simulink model "exp3_1_formation_linear"  (R2020b)
settings: Solver=VariableStepAuto  StartTime=0  StopTime=50  RelTol=1e-3
values from neighbouring files (symbols this model uses):
  g = 9.8    [run_exp1.m]    (also in run_exp2.m; run_exp3_1.m; run_exp3_2.m)
  Ixx = 0.114    [run_exp1.m]    (also in run_exp2.m; run_exp3_1.m; run_exp3_2.m)
  Iyy = 0.114    [run_exp1.m]    (also in run_exp2.m; run_exp3_1.m; run_exp3_2.m)
  Izz = 0.158    [run_exp1.m]    (also in run_exp2.m; run_exp3_1.m; run_exp3_2.m)
  k_F = 6.11*10^(-8)*3600/(4*pi^2)    (= 5.57165188849e-06)    [run_exp1.m]    (also in run_exp2.m; run_exp3_1.m; run_exp3_2.m)
  k_M = 1.5*10^(-9)*3600/(4*pi^2)    (= 1.36783597917e-07)    [run_exp1.m]    (also in run_exp2.m; run_exp3_1.m; run_exp3_2.m)
  k_m = 20    [run_exp1.m]    (also in run_exp2.m; run_exp3_1.m; run_exp3_2.m)
  kat_i = 0.05    [run_exp2.m]    (also in run_exp3_1.m; run_exp3_2.m)
  kat_p = 1    [run_exp2.m]    (also in run_exp3_1.m; run_exp3_2.m)
  kct_d = 1    [run_exp2.m]    (also in run_exp3_1.m; run_exp3_2.m)
  kct_i = 0.05    [run_exp2.m]    (also in run_exp3_1.m; run_exp3_2.m)
  kct_p = 1    [run_exp2.m]    (also in run_exp3_1.m; run_exp3_2.m)
  kd_phi = 4000    [run_exp1.m]    (also in run_exp2.m; run_exp3_1.m; run_exp3_2.m)
  kd_psi = 4000    [run_exp1.m]    (also in run_exp2.m; run_exp3_1.m; run_exp3_2.m)
  kd_theta = 4000    [run_exp1.m]    (also in run_exp2.m; run_exp3_1.m; run_exp3_2.m)
  kd_x = 1.0    (= 1)    [run_exp1.m]    (also in run_exp2.m; run_exp3_1.m; run_exp3_2.m)
  kd_y = 1.0    (= 1)    [run_exp1.m]    (also in run_exp2.m; run_exp3_1.m; run_exp3_2.m)
  kd_z = 2.0    (= 2)    [run_exp1.m]    (also in run_exp2.m; run_exp3_1.m; run_exp3_2.m)
  ki_x = 3e-4    (= 0.0003)    [run_exp1.m]    (also in run_exp2.m; run_exp3_1.m; run_exp3_2.m = 0.01)
  ki_y = 3e-4    (= 0.0003)    [run_exp1.m]    (also in run_exp2.m; run_exp3_1.m; run_exp3_2.m = 0.01)
  ki_z = 1e-6    (= 1e-06)    [run_exp1.m]    (also in run_exp2.m; run_exp3_1.m; run_exp3_2.m)
  kp_phi = 2000    [run_exp1.m]    (also in run_exp2.m; run_exp3_1.m; run_exp3_2.m)
  kp_psi = 800    [run_exp1.m]    (also in run_exp2.m; run_exp3_1.m; run_exp3_2.m)
  kp_theta = 2000    [run_exp1.m]    (also in run_exp2.m; run_exp3_1.m; run_exp3_2.m)
  kp_x = 0.5    [run_exp1.m]    (also in run_exp2.m; run_exp3_1.m; run_exp3_2.m = 1)
  kp_y = 0.5    [run_exp1.m]    (also in run_exp2.m; run_exp3_1.m; run_exp3_2.m = 1)
  kp_z = 1.2    [run_exp1.m]    (also in run_exp2.m; run_exp3_1.m; run_exp3_2.m)
  L = 0.2    [run_exp1.m]    (also in run_exp2.m; run_exp3_1.m; run_exp3_2.m)
  m = 0.5    [run_exp1.m]    (also in run_exp2.m; run_exp3_1.m; run_exp3_2.m)
  R = 0.5    [run_exp3_1.m]    (also in run_exp3_2.m = formation(4))
  state_track = [0,0,0,0 ... (first row only)    [run_exp2.m]    (also in run_exp3_1.m)
  y1_init = 0    [run_exp3_1.m]    (also in run_exp3_2.m)
  y2_init = R    (= 0.5)    [run_exp3_1.m]    (also in run_exp3_2.m = 5)
  y3_init = -R    (= -0.5)    [run_exp3_1.m]    (also in run_exp3_2.m = -5)
libraries: pid_lib x12, shared6dof x3, dspindex x1, dspswit3 x1
(part 2 of 2)

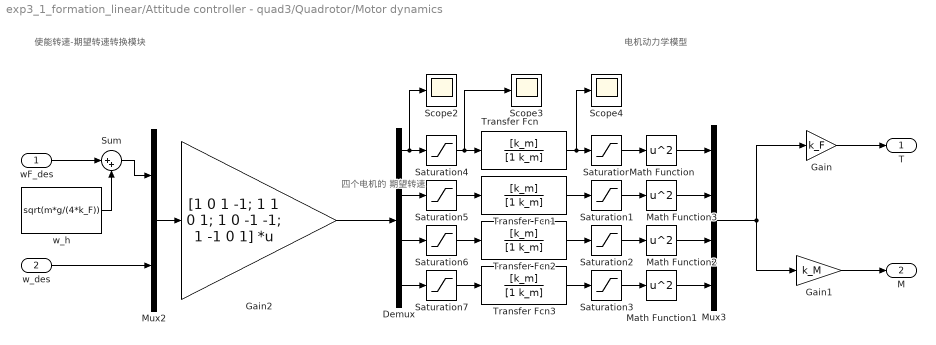
== system exp3_1_formation_linear/Attitude controller - quad3/Quadrotor/Motor dynamics ==
  note: 四个电机的
      | 期望转速
  note: 电机动力学模型
  note: 使能转速-期望转速转换模块
  wF_des : Inport
  w_des : Inport  Port=2
  Demux : Demux
  Gain : Gain  Gain=k_F
  Gain1 : Gain  Gain=k_M
  Gain2 : Gain  Gain=[1 0 1 -1; 1 1 0 1; 1 0 -1 -1; 1 -1 0 1]  Multiplication=Matrix(K*u) (u vector)
  Math Function{,1..3} (4 alike) : Math  Operator=square  SaturateOnIntegerOverflow=on
  Mux2 : Mux  Inputs=2
  Mux3 : Mux
  Saturation{,1..7} (8 alike) : Saturate  UpperLimit=7800*2*pi/60  LowerLimit=1200*2*pi/60
  Scope2 : Scope
  Scope3 : Scope
  Scope4 : Scope
  Sum : Sum  Inputs=|++
  Transfer Fcn{,1..3} (4 alike) : TransferFcn  Numerator=[k_m]  Denominator=[1 k_m]
  w_h : Constant  Value=sqrt(m*g/(4*k_F))
  T : Outport
  M : Outport  Port=2
  wires:
  Mux2/1 -> Gain2/1
  Sum/1 -> Mux2/1
  w_h/1 -> Sum/2
  Gain/1 -> T/1
  Mux3/1 -> Gain1/1, Gain/1
  Gain2/1 -> Demux/1
  Gain1/1 -> M/1
  wF_des/1 -> Sum/1
  Math Function/1 -> Mux3/1
  Math Function3/1 -> Mux3/2
  Math Function2/1 -> Mux3/3
  Math Function1/1 -> Mux3/4
  Transfer Fcn3/1 -> Saturation3/1
  Transfer Fcn/1 -> Scope4/1, Saturation/1
  Transfer Fcn1/1 -> Saturation1/1
  Transfer Fcn2/1 -> Saturation2/1
  Saturation/1 -> Math Function/1
  Saturation3/1 -> Math Function1/1
  Saturation2/1 -> Math Function2/1
  Saturation1/1 -> Math Function3/1
  w_des/1 -> Mux2/2
  Saturation6/1 -> Transfer Fcn2/1
  Saturation7/1 -> Transfer Fcn3/1
  Saturation4/1 -> Scope3/1, Transfer Fcn/1
  Saturation5/1 -> Transfer Fcn1/1
  Demux/1 -> Scope2/1, Saturation4/1
  Demux/2 -> Saturation5/1
  Demux/3 -> Saturation6/1
  Demux/4 -> Saturation7/1

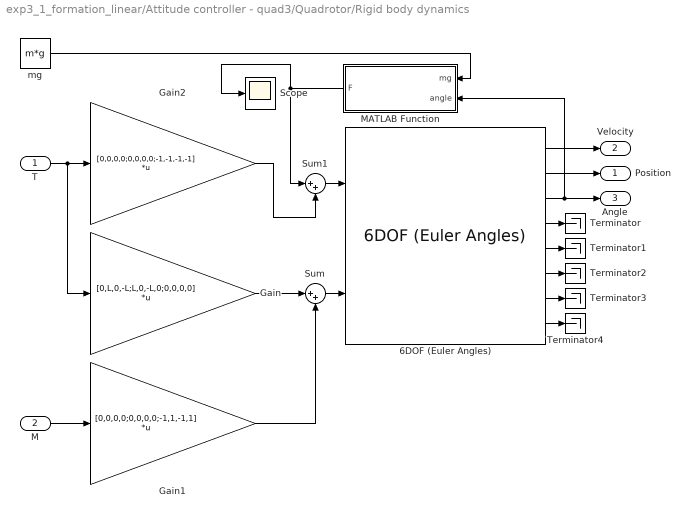
== system exp3_1_formation_linear/Attitude controller - quad3/Quadrotor/Rigid body dynamics ==
  T : Inport
  M : Inport  Port=2
  6DOF (Euler Angles) : shared6dof/6DOF (Euler Angles)  units=Metric (MKS)  mtype=Fixed  rep=Euler Angles  xme_0=[0 y3_init 0]  Vm_0=[0 0 0]  eul_0=[0 0 0]  pm_0=[0 0 0]  mass_0=m  mass_e=0.5  mass_f=2.0  inertia=[Ixx,0,0; 0,Iyy,0; 0,0,Izz]  inertia_e=eye(3)  inertia_f=2*eye(3)  k_quat=1.0  vre_flag=on  abi_flag=off  aMode=0  xme_statename=''  Vm_statename=''  eul_statename=''  quat_statename=''  pm_statename=''  mass_statename=''
      settings: SourceProductBaseCode=AE,PW,MT,UV,VE,VP
  Gain : Gain  Gain=[0,L,0,-L;L,0,-L,0;0,0,0,0]  Multiplication=Matrix(K*u) (u vector)
  Gain1 : Gain  Gain=[0,0,0,0;0,0,0,0;-1,1,-1,1]  Multiplication=Matrix(K*u) (u vector)
  Gain2 : Gain  Gain=[0,0,0,0;0,0,0,0;-1,-1,-1,-1]  Multiplication=Matrix(K*u) (u vector)
  MATLAB Function : MATLAB Function  TreatAsAtomicUnit=on
  Scope : Scope
  Sum : Sum  Inputs=|++
  Sum1 : Sum  Inputs=|++
  Terminator{,1..4} (5 alike) : Terminator
  mg : Constant  Value=m*g
  Position : Outport
  Velocity : Outport  Port=2
  Angle : Outport  Port=3
  wires:
  6DOF (Euler Angles)/1 -> Velocity/1
  T/1 -> Gain/1, Gain2/1
  6DOF (Euler Angles)/3 -> MATLAB Function/2(angle), Angle/1
  6DOF (Euler Angles)/2 -> Position/1
  Gain1/1 -> Sum/2
  Gain/1 -> Sum/1
  Sum/1 -> 6DOF (Euler Angles)/2
  M/1 -> Gain1/1
  Sum1/1 -> 6DOF (Euler Angles)/1
  Gain2/1 -> Sum1/2
  6DOF (Euler Angles)/4 -> Terminator/1
  6DOF (Euler Angles)/5 -> Terminator1/1
  6DOF (Euler Angles)/6 -> Terminator2/1
  6DOF (Euler Angles)/7 -> Terminator3/1
  6DOF (Euler Angles)/8 -> Terminator4/1
  mg/1 -> MATLAB Function/1(mg)
  MATLAB Function/1(F) -> Sum1/1, Scope/1

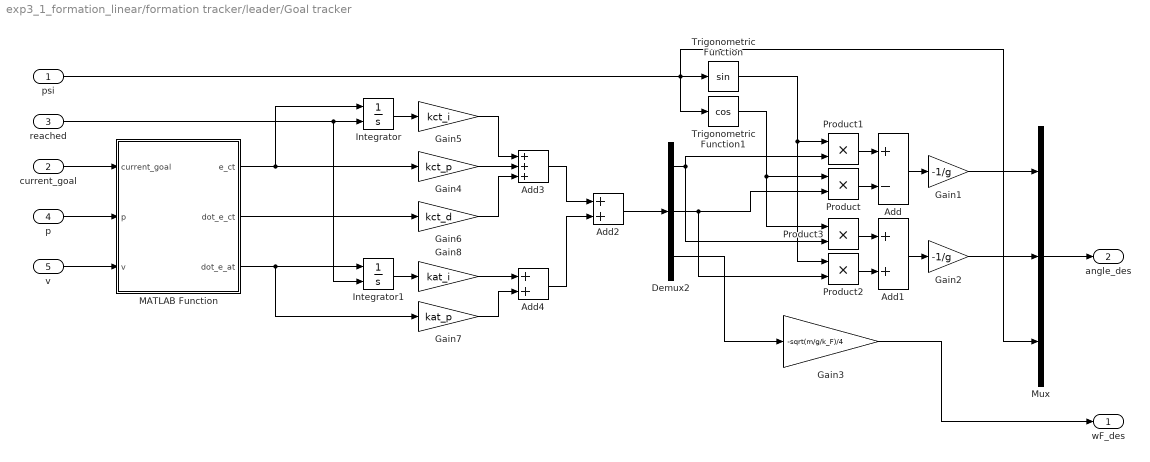
== system exp3_1_formation_linear/formation tracker/leader/Goal tracker ==
  psi : Inport
  current_goal : Inport  Port=2
  reached : Inport  Port=3
  p : Inport  Port=4
  v : Inport  Port=5
  Add : Sum  Inputs=+-
  Add1 : Sum
  Add2 : Sum
  Add3 : Sum  Inputs=+++
  Add4 : Sum
  Demux2 : Demux  Outputs=3
  Gain1 : Gain  Gain=-1/g
  Gain2 : Gain  Gain=-1/g
  Gain3 : Gain  Gain=-sqrt(m/g/k_F)/4
  Gain4 : Gain  Gain=kct_p
  Gain5 : Gain  Gain=kct_i
  Gain6 : Gain  Gain=kct_d
  Gain7 : Gain  Gain=kat_p
  Gain8 : Gain  Gain=kat_i
  Integrator : Integrator  ExternalReset=rising
  Integrator1 : Integrator  ExternalReset=rising
  MATLAB Function : MATLAB Function  TreatAsAtomicUnit=on
  Mux : Mux  Inputs=3
  Product{,1..3} (4 alike) : Product
  Trigonometric Function : Trigonometry
  Trigonometric Function1 : Trigonometry  Operator=cos
  wF_des : Outport
  angle_des : Outport  Port=2
  wires:
  Mux/1 -> angle_des/1
  Gain2/1 -> Mux/2
  Add4/1 -> Add2/2
  Add2/1 -> Demux2/1
  Trigonometric Function1/1 -> Product3/1, Product/1
  MATLAB Function/1(e_ct) -> Integrator/1, Gain4/1
  Demux2/1 -> Product3/2, Product1/2
  psi/1 -> Mux/3, Trigonometric Function1/1, Trigonometric Function/1
  Gain6/1 -> Add3/3
  Add3/1 -> Add2/1
  Product2/1 -> Add1/2
  Trigonometric Function/1 -> Product2/1, Product1/1
  reached/1 -> Integrator1/2, Integrator/2
  Product/1 -> Add/2
  Gain1/1 -> Mux/1
  Demux2/2 -> Product2/2, Product/2
  Demux2/3 -> Gain3/1
  Product3/1 -> Add1/1
  Add/1 -> Gain1/1
  v/1 -> MATLAB Function/3(v)
  Product1/1 -> Add/1
  MATLAB Function/3(dot_e_at) -> Gain7/1, Integrator1/1
  Integrator/1 -> Gain5/1
  Gain5/1 -> Add3/1
  Gain8/1 -> Add4/1
  Integrator1/1 -> Gain8/1
  Gain7/1 -> Add4/2
  Gain4/1 -> Add3/2
  Add1/1 -> Gain2/1
  current_goal/1 -> MATLAB Function/1(current_goal)
  MATLAB Function/2(dot_e_ct) -> Gain6/1
  p/1 -> MATLAB Function/2(p)
  Gain3/1 -> wF_des/1

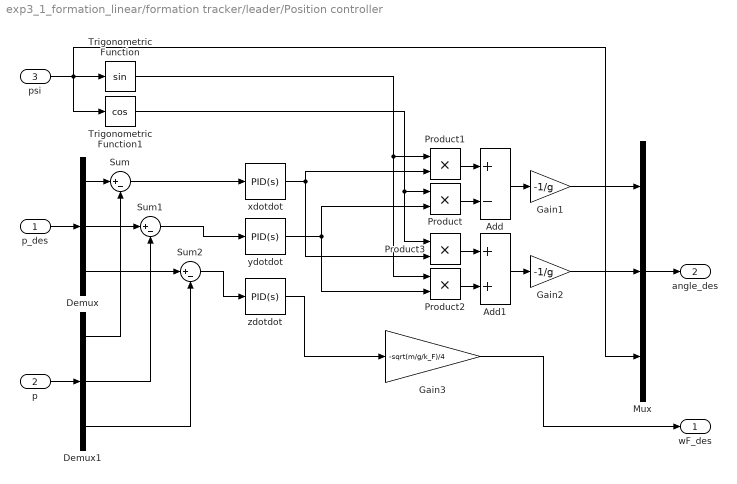
== system exp3_1_formation_linear/formation tracker/leader/Position controller ==
  p_des : Inport
  p : Inport  Port=2
  psi : Inport  Port=3
  Add : Sum  Inputs=+-
  Add1 : Sum
  Demux : Demux  Outputs=3
  Demux1 : Demux  Outputs=3
  Gain1 : Gain  Gain=-1/g
  Gain2 : Gain  Gain=-1/g
  Gain3 : Gain  Gain=-sqrt(m/g/k_F)/4
  Mux : Mux  Inputs=3
  Product{,1..3} (4 alike) : Product
  Sum : Sum  Inputs=|+-
  Sum1 : Sum  Inputs=|+-
  Sum2 : Sum  Inputs=|+-
  Trigonometric Function : Trigonometry
  Trigonometric Function1 : Trigonometry  Operator=cos
  xdotdot : pid_lib/PID Controller  Controller=PID  Form=Parallel  TimeDomain=Continuous-time  UseExternalTs=off  SampleTime=-1  IntegratorMethod=Forward Euler  FilterMethod=Forward Euler  ControllerParametersSource=internal  P=kp_x  I=ki_x  D=kd_x  UseFilter=on  N=100  TunerSelectOption=Transfer Function Based (PID Tuner App)  InitialConditionSource=internal  InitialConditionForIntegrator=0  InitialConditionForFilter=0  DifferentiatorICPrevScaledInput=0  ExternalReset=none  TrackingMode=off  Kt=1  LimitOutput=off  SatLimitsSource=internal  UpperSaturationLimit=inf  LowerSaturationLimit=-inf  LinearizeAsGain=on  AntiWindupMode=none  Kb=1  POutMin=[]  POutMax=[]  IOutMin=[]  IOutMax=[]  DOutMin=[]  DOutMax=[]  NOutMin=[]  NOutMax=[]  SumOutMin=[]  SumOutMax=[]  SaturationOutMin=[]  SaturationOutMax=[]  PParamMin=[]  PParamMax=[]  IParamMin=[]  IParamMax=[]  DParamMin=[]  DParamMax=[]  NParamMin=[]  NParamMax=[]  KbParamMin=[]  KbParamMax=[]  KtParamMin=[]  KtParamMax=[]  KbOutMin=[]  KbOutMax=[]  KtOutMin=[]  KtOutMax=[]  IntegratorOutMin=[]  IntegratorOutMax=[]  FilterOutMin=[]  FilterOutMax=[]  SumI1OutMin=[]  SumI1OutMax=[]  SumI2OutMin=[]  SumI2OutMax=[]  SumI3OutMin=[]  SumI3OutMax=[]  SumI4OutMin=[]  SumI4OutMax=[]  SumDOutMin=[]  SumDOutMax=[]  DifferentiatorOutMin=[]  DifferentiatorOutMax=[]  FilterDiffOutCoefMin=[]  FilterDiffOutCoefMax=[]  ReciprocalOutMin=[]  ReciprocalOutMax=[]  SumDenOutMin=[]  SumDenOutMax=[]  SumNumOutMin=[]  SumNumOutMax=[]  DivideOutMin=[]  DivideOutMax=[]  UdiffTsProdOutMin=[]  UdiffTsProdOutMax=[]  NTsProdOutMin=[]  NTsProdOutMax=[]  UintegralTsProdOutMin=[]  UintegralTsProdOutMax=[]  UngainTsProdOutMin=[]  UngainTsProdOutMax=[]  IntegratorContinuousStateAttributes=''  IntegratorStateMustResolveToSignalObject=off  IntegratorRTWStateStorageClass=Auto  FilterContinuousStateAttributes=''  FilterStateMustResolveToSignalObject=off  FilterRTWStateStorageClass=Auto  ParallelPVariant=InternalParameters  IdealPVariant=Disabled  IVariant=InternalParameters  DVariant=InternalParameters  IntegratorVariant=Continuous  SatVariant=Disabled  AWVariant=Passthrough  PCopyVariant=Disabled  TRVariant=Disabled  FdbkBlocksVariant=Forward  IdealPFdbkVariant=Disabled  SatFdbkVariant=Disabled  DerivativeFilterVariant=ContFilter  NVariant=InternalParameters  NCopyVariant=Disabled  FilterICVariant=InternalICsFilter  IntegratorICVariant=InternalICs  ExternalResetVariant=Disabled  TRSumVariant=Passthrough  SumFdbkVariant=Disabled  SumVariant=Sum_PID  TsampFilterVariant=InternalTs  TsampNgainVariant=Passthrough  TsampIntegralVariant=Passthrough  ExternalSaturationOutDataTypeStr=Inherit: Same as second input
  ydotdot : pid_lib/PID Controller  Controller=PID  Form=Parallel  TimeDomain=Continuous-time  UseExternalTs=off  SampleTime=-1  IntegratorMethod=Forward Euler  FilterMethod=Forward Euler  ControllerParametersSource=internal  P=kp_y  I=ki_y  D=kd_y  UseFilter=on  N=100  TunerSelectOption=Transfer Function Based (PID Tuner App)  InitialConditionSource=internal  InitialConditionForIntegrator=0  InitialConditionForFilter=0  DifferentiatorICPrevScaledInput=0  ExternalReset=none  TrackingMode=off  Kt=1  LimitOutput=off  SatLimitsSource=internal  UpperSaturationLimit=inf  LowerSaturationLimit=-inf  LinearizeAsGain=on  AntiWindupMode=none  Kb=1  POutMin=[]  POutMax=[]  IOutMin=[]  IOutMax=[]  DOutMin=[]  DOutMax=[]  NOutMin=[]  NOutMax=[]  SumOutMin=[]  SumOutMax=[]  SaturationOutMin=[]  SaturationOutMax=[]  PParamMin=[]  PParamMax=[]  IParamMin=[]  IParamMax=[]  DParamMin=[]  DParamMax=[]  NParamMin=[]  NParamMax=[]  KbParamMin=[]  KbParamMax=[]  KtParamMin=[]  KtParamMax=[]  KbOutMin=[]  KbOutMax=[]  KtOutMin=[]  KtOutMax=[]  IntegratorOutMin=[]  IntegratorOutMax=[]  FilterOutMin=[]  FilterOutMax=[]  SumI1OutMin=[]  SumI1OutMax=[]  SumI2OutMin=[]  SumI2OutMax=[]  SumI3OutMin=[]  SumI3OutMax=[]  SumI4OutMin=[]  SumI4OutMax=[]  SumDOutMin=[]  SumDOutMax=[]  DifferentiatorOutMin=[]  DifferentiatorOutMax=[]  FilterDiffOutCoefMin=[]  FilterDiffOutCoefMax=[]  ReciprocalOutMin=[]  ReciprocalOutMax=[]  SumDenOutMin=[]  SumDenOutMax=[]  SumNumOutMin=[]  SumNumOutMax=[]  DivideOutMin=[]  DivideOutMax=[]  UdiffTsProdOutMin=[]  UdiffTsProdOutMax=[]  NTsProdOutMin=[]  NTsProdOutMax=[]  UintegralTsProdOutMin=[]  UintegralTsProdOutMax=[]  UngainTsProdOutMin=[]  UngainTsProdOutMax=[]  IntegratorContinuousStateAttributes=''  IntegratorStateMustResolveToSignalObject=off  IntegratorRTWStateStorageClass=Auto  FilterContinuousStateAttributes=''  FilterStateMustResolveToSignalObject=off  FilterRTWStateStorageClass=Auto  ParallelPVariant=InternalParameters  IdealPVariant=Disabled  IVariant=InternalParameters  DVariant=InternalParameters  IntegratorVariant=Continuous  SatVariant=Disabled  AWVariant=Passthrough  PCopyVariant=Disabled  TRVariant=Disabled  FdbkBlocksVariant=Forward  IdealPFdbkVariant=Disabled  SatFdbkVariant=Disabled  DerivativeFilterVariant=ContFilter  NVariant=InternalParameters  NCopyVariant=Disabled  FilterICVariant=InternalICsFilter  IntegratorICVariant=InternalICs  ExternalResetVariant=Disabled  TRSumVariant=Passthrough  SumFdbkVariant=Disabled  SumVariant=Sum_PID  TsampFilterVariant=InternalTs  TsampNgainVariant=Passthrough  TsampIntegralVariant=Passthrough  ExternalSaturationOutDataTypeStr=Inherit: Same as second input
  zdotdot : pid_lib/PID Controller  Controller=PID  Form=Parallel  TimeDomain=Continuous-time  UseExternalTs=off  SampleTime=-1  IntegratorMethod=Forward Euler  FilterMethod=Forward Euler  ControllerParametersSource=internal  P=kp_z  I=ki_z  D=kd_z  UseFilter=on  N=100  TunerSelectOption=Transfer Function Based (PID Tuner App)  InitialConditionSource=internal  InitialConditionForIntegrator=0  InitialConditionForFilter=0  DifferentiatorICPrevScaledInput=0  ExternalReset=none  TrackingMode=off  Kt=1  LimitOutput=off  SatLimitsSource=internal  UpperSaturationLimit=inf  LowerSaturationLimit=-inf  LinearizeAsGain=on  AntiWindupMode=none  Kb=1  POutMin=[]  POutMax=[]  IOutMin=[]  IOutMax=[]  DOutMin=[]  DOutMax=[]  NOutMin=[]  NOutMax=[]  SumOutMin=[]  SumOutMax=[]  SaturationOutMin=[]  SaturationOutMax=[]  PParamMin=[]  PParamMax=[]  IParamMin=[]  IParamMax=[]  DParamMin=[]  DParamMax=[]  NParamMin=[]  NParamMax=[]  KbParamMin=[]  KbParamMax=[]  KtParamMin=[]  KtParamMax=[]  KbOutMin=[]  KbOutMax=[]  KtOutMin=[]  KtOutMax=[]  IntegratorOutMin=[]  IntegratorOutMax=[]  FilterOutMin=[]  FilterOutMax=[]  SumI1OutMin=[]  SumI1OutMax=[]  SumI2OutMin=[]  SumI2OutMax=[]  SumI3OutMin=[]  SumI3OutMax=[]  SumI4OutMin=[]  SumI4OutMax=[]  SumDOutMin=[]  SumDOutMax=[]  DifferentiatorOutMin=[]  DifferentiatorOutMax=[]  FilterDiffOutCoefMin=[]  FilterDiffOutCoefMax=[]  ReciprocalOutMin=[]  ReciprocalOutMax=[]  SumDenOutMin=[]  SumDenOutMax=[]  SumNumOutMin=[]  SumNumOutMax=[]  DivideOutMin=[]  DivideOutMax=[]  UdiffTsProdOutMin=[]  UdiffTsProdOutMax=[]  NTsProdOutMin=[]  NTsProdOutMax=[]  UintegralTsProdOutMin=[]  UintegralTsProdOutMax=[]  UngainTsProdOutMin=[]  UngainTsProdOutMax=[]  IntegratorContinuousStateAttributes=''  IntegratorStateMustResolveToSignalObject=off  IntegratorRTWStateStorageClass=Auto  FilterContinuousStateAttributes=''  FilterStateMustResolveToSignalObject=off  FilterRTWStateStorageClass=Auto  ParallelPVariant=InternalParameters  IdealPVariant=Disabled  IVariant=InternalParameters  DVariant=InternalParameters  IntegratorVariant=Continuous  SatVariant=Disabled  AWVariant=Passthrough  PCopyVariant=Disabled  TRVariant=Disabled  FdbkBlocksVariant=Forward  IdealPFdbkVariant=Disabled  SatFdbkVariant=Disabled  DerivativeFilterVariant=ContFilter  NVariant=InternalParameters  NCopyVariant=Disabled  FilterICVariant=InternalICsFilter  IntegratorICVariant=InternalICs  ExternalResetVariant=Disabled  TRSumVariant=Passthrough  SumFdbkVariant=Disabled  SumVariant=Sum_PID  TsampFilterVariant=InternalTs  TsampNgainVariant=Passthrough  TsampIntegralVariant=Passthrough  ExternalSaturationOutDataTypeStr=Inherit: Same as second input
  wF_des : Outport
  angle_des : Outport  Port=2
  wires:
  Demux/1 -> Sum/1
  Demux/2 -> Sum1/1
  Demux/3 -> Sum2/1
  Sum/1 -> xdotdot/1
  Demux1/2 -> Sum1/2
  Demux1/3 -> Sum2/2
  Demux1/1 -> Sum/2
  p_des/1 -> Demux/1
  p/1 -> Demux1/1
  Sum1/1 -> ydotdot/1
  Sum2/1 -> zdotdot/1
  psi/1 -> Trigonometric Function1/1, Mux/3, Trigonometric Function/1
  Mux/1 -> angle_des/1
  Gain1/1 -> Mux/1
  Add/1 -> Gain1/1
  Product1/1 -> Add/1
  Product/1 -> Add/2
  Product2/1 -> Add1/2
  Product3/1 -> Add1/1
  Add1/1 -> Gain2/1
  xdotdot/1 -> Product3/2, Product1/2
  Trigonometric Function/1 -> Product2/1, Product1/1
  ydotdot/1 -> Product2/2, Product/2
  Trigonometric Function1/1 -> Product3/1, Product/1
  Gain2/1 -> Mux/2
  zdotdot/1 -> Gain3/1
  Gain3/1 -> wF_des/1

== system exp3_1_formation_linear/formation tracker/leader/update current goal ==
  state_track : Inport
  position : Inport  Port=2
  Counter : dspswit3/Counter  Direction=Up  CountEvent=Rising edge  CounterSize=User defined  MaxCount=255  InitialCount=0  Output=Count  HitValue=32  ResetInput=off  SamplesPerFrame=1  Ts=1  CntDtype=double  HitDtype=Logical
  MATLAB Function : MATLAB Function  TreatAsAtomicUnit=on
  MATLAB Function1 : MATLAB Function  TreatAsAtomicUnit=on
  MATLAB Function2 : MATLAB Function  TreatAsAtomicUnit=on
  Relational Operator : RelationalOperator  OutDataTypeStr=boolean  RndMeth=Simplest
  current_goal : Outport
  reached : Outport  Port=2
  Finished : Outport  Port=3
  wires:
  Relational Operator/1 -> Finished/1
  MATLAB Function1/1(current_goal) -> MATLAB Function2/1(current_goal), current_goal/1
  Counter/1 -> Relational Operator/1, MATLAB Function1/2(cnt), reached/1
  state_track/1 -> MATLAB Function/1(state_track)
  MATLAB Function/2(max_num) -> Relational Operator/2
  MATLAB Function2/1(flag) -> Counter/1
  position/1 -> MATLAB Function2/2(position)
  MATLAB Function/1(full_state) -> MATLAB Function1/1(full_state)

== matlab function exp3_1_formation_linear/formation tracker/follower_des2 ==
  data: ref input; p_des_follower output
function p_des_follower = p_des_follower1(ref)
leader_p = ref(1:3);
leader_v = ref(4:6);
R = ref(end); % R为编队距离

if norm([leader_v(1),leader_v(2)])==0
    dir = [0;-1;0];
else
    dir = [leader_v(2);-leader_v(1);0];
end

uni_dir = dir/norm(dir);

p_des_follower = leader_p + R*uni_dir;

end

== matlab function exp3_1_formation_linear/Attitude controller - quad1/Quadrotor/Rigid body dynamics/MATLAB Function ==
  data: mg input; angle input; F output
function F = mg_w2b(mg, angle)
phi = angle(1);
theta = angle(2);
F = [-sin(theta);cos(theta)*sin(phi);cos(phi)*cos(theta)] * mg;
end

== matlab function exp3_1_formation_linear/formation tracker/follower_des1 ==
  data: ref input; p_des_follower output
function p_des_follower = p_des_follower1(ref)
leader_p = ref(1:3);
leader_v = ref(4:6);
R = ref(end); % R为编队距离

if norm([leader_v(1),leader_v(2)])==0
    dir = [0;1;0];
else
    dir = [-leader_v(2);leader_v(1);0];
end

uni_dir = dir/norm(dir);

p_des_follower = leader_p + R*uni_dir;

end

== matlab function exp3_1_formation_linear/Attitude controller - quad2/Quadrotor/Rigid body dynamics/MATLAB Function ==
  data: mg input; angle input; F output
function F = mg_w2b(mg, angle)
phi = angle(1);
theta = angle(2);
F = [-sin(theta);cos(theta)*sin(phi);cos(phi)*cos(theta)] * mg;
end

== matlab function exp3_1_formation_linear/Attitude controller - quad3/Quadrotor/Rigid body dynamics/MATLAB Function ==
  data: mg input; angle input; F output
function F = mg_w2b(mg, angle)
phi = angle(1);
theta = angle(2);
F = [-sin(theta);cos(theta)*sin(phi);cos(phi)*cos(theta)] * mg;
end

== matlab function exp3_1_formation_linear/formation tracker/leader/Goal tracker/MATLAB Function ==
  data: current_goal input; e_ct output; p input; v input; dot_e_ct output; dot_e_at output
function [e_ct,dot_e_ct,dot_e_at] = get_error(current_goal,p,v)
% current_goal是列向量
p_des = current_goal(1:3); % 期望位置，此处是尚未到达的航点
ti = current_goal(4:6); % 方向向量
v_des = current_goal(7)*ti; % 速度向量

e_ct = (p - p_des)'*ti.*ti - (p - p_des);
dot_e_ct = (v'*ti).*ti - v;
dot_e_at = v_des - (v'*ti).*ti;
end

== matlab function exp3_1_formation_linear/formation tracker/leader/update current goal/MATLAB Function ==
  data: state_track input; full_state output; max_num output
function [full_state,max_num] = load_state(state_track)
% 将来自工作空间的state_track(n*4)，转换为(n*7):[[x,y,z],[ti_x,ti_y,ti_z]（指向该点的方向向量）,v]
n = size(state_track,1); % 航路点数，含起始点
full_state = zeros(n-1,7); % 期望状态点序列（不含起始点）
for i = 1:n-1
    uni_vector = (state_track(i+1,1:3) - state_track(i,1:3) ) / norm(state_track(i+1,1:3) - state_track(i,1:3));
    full_state(i,:) = [state_track(i+1,1:3), uni_vector, state_track(i+1,4)];
end
max_num = n-1; % 目标点数量，不含起始点

end

== matlab function exp3_1_formation_linear/formation tracker/leader/update current goal/MATLAB Function1 ==
  data: full_state input; current_goal output; cnt input
function current_goal = get_current_goal(full_state, cnt)
% 以cnt为索引，输出此时期望的state
current_goal = full_state(min(round(cnt)+1,size(full_state,1)),:)';
end

== matlab function exp3_1_formation_linear/formation tracker/leader/update current goal/MATLAB Function2 ==
  data: current_goal input; position input; flag output
function flag = reached_current_goal(current_goal,position)
% 对比当前位置与目标位置，如果足够接近，则认为到达了目标位置，输出1
threshold = 1;
flag = norm(position-current_goal(1:3)) < threshold;
end
